simulink model "AIN_3x_3VT"  (R2018b)
settings: Solver=ode23t  StartTime=0.0  StopTime=0.5  RelTol=1e-3
undefined symbols (not defined in the file): DiscIntNeverNeededParam, fout
libraries: powerlib x26, powerlib_meascontrol x4
settings Model: Creator=K2  LastModifiedBy=VID Company

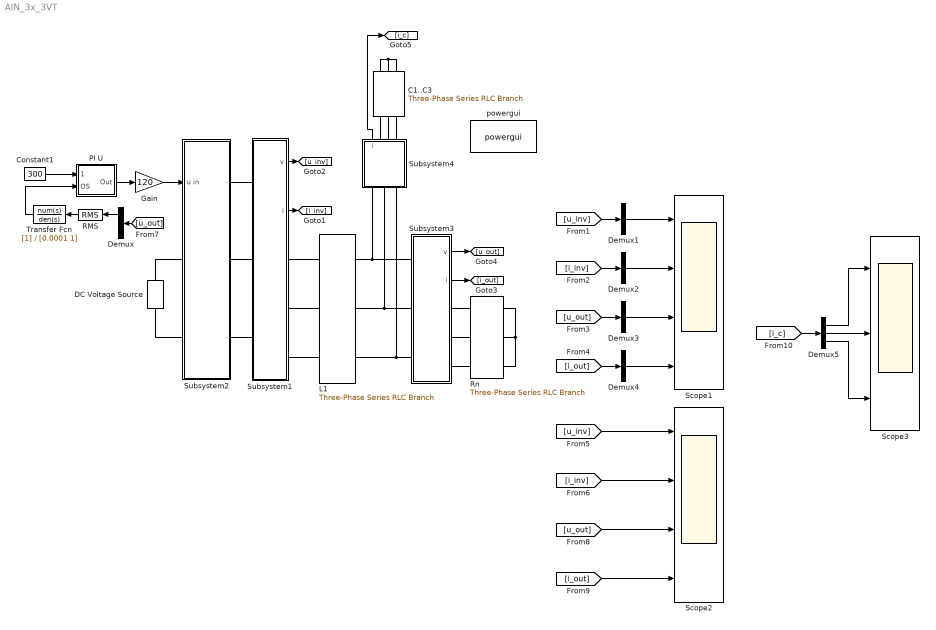
== system AIN_3x_3VT ==
  C1..C3 : powerlib/Elements/Three-Phase Series RLC Branch  LConnTagsString=A|B|C  RConnTagsString=A|B|C  BranchType=RC  Resistance=0.020  Inductance=1e-3  Capacitance=20e-6  Measurements=None
  Constant1 : Constant  Value=300  SampleTime=1e-6
  DC Voltage Source : powerlib/Electrical Sources/DC Voltage Source  Amplitude=550  Measurements=None
  Demux{,1..5} (6 alike) : Demux  Outputs=3
  Gain : Gain  Gain=120
  L1 : powerlib/Elements/Three-Phase Series RLC Branch  LConnTagsString=A|B|C  RConnTagsString=A|B|C  BranchType=RL  Resistance=0.2  Inductance=0.5e-3  Capacitance=1e-6  Measurements=None
  PI U : Subsystem
  RMS : powerlib_meascontrol/Measurements/RMS  TrueRMS=off  Freq=fout  RMSInit=0  Ts=0
  Rn : powerlib/Elements/Three-Phase Series RLC Branch  LConnTagsString=A|B|C  RConnTagsString=A|B|C  BranchType=RL  Resistance=10/sqrt(3)  Inductance=0.01e-3  Capacitance=1e-6  Measurements=None
  Scope1 : Scope  NumInputPorts=4
  Scope2 : Scope  NumInputPorts=4
  Scope3 : Scope  NumInputPorts=3
  Subsystem1 : Subsystem
  Subsystem2 : Subsystem
  Subsystem3 : Subsystem
  Subsystem4 : Subsystem
  Transfer Fcn : TransferFcn  Denominator=[0.0001 1]
  powergui : powerlib/powergui  Priority=1  SimulationMode=Discrete  SampleTime=1e-7  frequency=60  Iterations=50  frequencyindice=0  Pbase=100e6  ErrMax=1e-4  UnitsV=kV  UnitsW=MW  buscounter=0  FunctionMessages=off  echomessages=off  EnableUseOfTLC=off  CurrentSourceSwitches=off  DisableSnubberDevices=off  DisableRonSwitches=off  DisableVfSwitches=off  DisplayEquations=off  SolverType=Tustin/Backward Euler (TBE)  Interpol=off  ExternalGateDelay=off  methode=off  Ts=100  x0status=blocks  SPID=on  SwTol=0  HookPort=off  RestoreLinks=warning  ResistiveCurrentMeasurement=off  Frange=[0:2:500]  Ylog=off  Xlog=on  ShowGrid=off  save=off  variable=ZData  structure=logsout  ZoomFFT=on  StartTime=0.4  cycles=5  DisplayStyle=1  fundamental=50  FreqAxis=off  MaxFrequency=20000  frequencyindicesteady=1  RmsSteady=1  display=off
  wires:
  Constant1/1 -> PI U/1(Zad)
  RMS/1 -> Transfer Fcn/1
  Gain/1 -> Subsystem2/1(u in)
  PI U/1(Out) -> Gain/1
  Transfer Fcn/1 -> PI U/2(OS)
  Subsystem1/2(i) -> [i_inv]
  Subsystem1/1(v) -> [u_inv]
  Subsystem3/1(v) -> [u_out]
  Subsystem3/2(i) -> [i_out]
  [u_out] -> Demux/1
  Demux/1 -> RMS/1
  [u_inv] -> Demux1/1
  Demux1/2 -> Scope1/1
  [i_inv] -> Demux2/1
  Demux2/2 -> Scope1/2
  [u_out] -> Demux3/1
  Demux3/2 -> Scope1/3
  [i_out] -> Demux4/1
  Demux4/2 -> Scope1/4
  [u_inv] -> Scope2/1
  [i_inv] -> Scope2/2
  [i_out] -> Scope2/4
  [u_out] -> Scope2/3
  Subsystem4/1(i) -> [i_c]
  [i_c] -> Demux5/1
  Demux5/2 -> Scope3/2
  Demux5/1 -> Scope3/1
  Demux5/3 -> Scope3/3
  connections:
  Subsystem3/LConn1 -- Subsystem4/LConn1 -- L1/RConn1
  Subsystem3/LConn2 -- Subsystem4/LConn2 -- L1/RConn2
  Subsystem3/LConn3 -- Subsystem4/LConn3 -- L1/RConn3
  C1..C3/RConn1 -- C1..C3/RConn2 -- C1..C3/RConn3
  Rn/RConn1 -- Rn/RConn2 -- Rn/RConn3
  Subsystem2/RConn3 -- Subsystem1/LConn3
  Subsystem2/RConn1 -- Subsystem1/LConn1
  Subsystem2/RConn2 -- Subsystem1/LConn2
  Subsystem1/RConn1 -- L1/LConn1
  Subsystem1/RConn2 -- L1/LConn2
  Subsystem1/RConn3 -- L1/LConn3
  Subsystem3/RConn1 -- Rn/LConn1
  Subsystem3/RConn2 -- Rn/LConn2
  Subsystem3/RConn3 -- Rn/LConn3
  DC Voltage Source/RConn1 -- Subsystem2/LConn1
  DC Voltage Source/LConn1 -- Subsystem2/LConn2
  C1..C3/LConn1 -- Subsystem4/RConn1
  C1..C3/LConn2 -- Subsystem4/RConn2
  C1..C3/LConn3 -- Subsystem4/RConn3

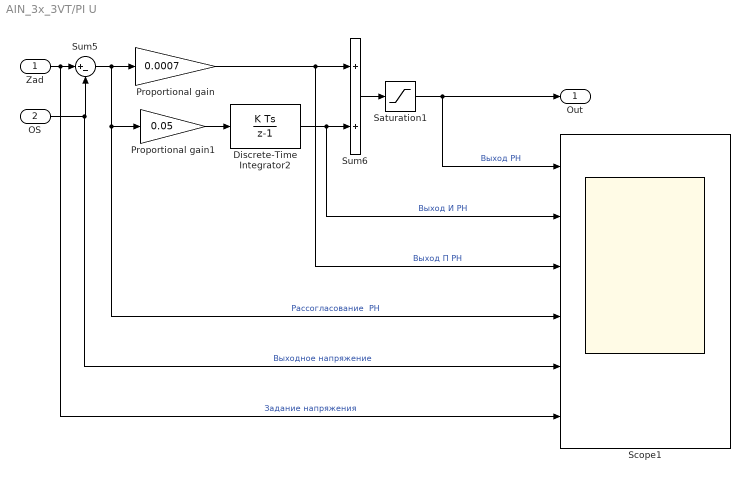
== system AIN_3x_3VT/PI U ==
  Zad : Inport
  OS : Inport  Port=2
  Discrete-Time Integrator2 : DiscreteIntegrator  SampleTime=-1  LimitOutput=on  UpperSaturationLimit=1  LowerSaturationLimit=0  ICPrevOutput=DiscIntNeverNeededParam  ICPrevScaledInput=DiscIntNeverNeededParam
  Proportional gain : Gain  Gain=0.0007  SaturateOnIntegerOverflow=on  OutDataTypeStr=Inherit: Same as input  ParamDataTypeStr=Inherit: Same as input
  Proportional gain1 : Gain  Gain=0.05  SaturateOnIntegerOverflow=on  OutDataTypeStr=Inherit: Same as input  ParamDataTypeStr=Inherit: Same as input
  Saturation1 : Saturate  UpperLimit=1  LowerLimit=0
  Scope1 : Scope  NumInputPorts=6
  Sum5 : Sum  Inputs=|+-  SaturateOnIntegerOverflow=on  InputSameDT=on  OutDataTypeStr=Inherit: Same as first input
  Sum6 : Sum  SaturateOnIntegerOverflow=on  InputSameDT=on  OutDataTypeStr=Inherit: Same as first input
  Out : Outport
  wires:
  Proportional gain/1 -> Scope1/3, Sum6/1  "Выход П РН"
  Discrete-Time Integrator2/1 -> Sum6/2, Scope1/2  "Выход И РН"
  OS/1 -> Scope1/5, Sum5/2  "Выходное напряжение"
  Zad/1 -> Scope1/6, Sum5/1  "Задание напряжения"
  Sum5/1 -> Proportional gain1/1, Scope1/4, Proportional gain/1  "Рассогласование  РН"
  Sum6/1 -> Saturation1/1
  Saturation1/1 -> Out/1, Scope1/1  "Выход РН"
  Proportional gain1/1 -> Discrete-Time Integrator2/1

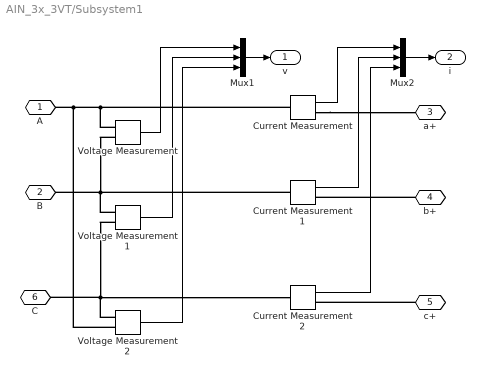
== system AIN_3x_3VT/Subsystem1 ==
  Current Measurement : powerlib/Measurements/Current Measurement  PhasorSimulation=off  OutputType=Complex  PSBequivalent=0
  Current Measurement1 : powerlib/Measurements/Current Measurement  PhasorSimulation=off  OutputType=Complex  PSBequivalent=0
  Current Measurement2 : powerlib/Measurements/Current Measurement  PhasorSimulation=off  OutputType=Complex  PSBequivalent=0
  Mux1 : Mux  Inputs=3
  Mux2 : Mux  Inputs=3
  Voltage Measurement : powerlib/Measurements/Voltage Measurement  PhasorSimulation=off  OutputType=Complex  PSBequivalent=0
  Voltage Measurement1 : powerlib/Measurements/Voltage Measurement  PhasorSimulation=off  OutputType=Complex  PSBequivalent=0
  Voltage Measurement2 : powerlib/Measurements/Voltage Measurement  PhasorSimulation=off  OutputType=Complex  PSBequivalent=0
  A : PMIOPort  Side=Left
  B : PMIOPort  Port=2  Side=Left
  a+ : PMIOPort  Port=3  Side=Right
  b+ : PMIOPort  Port=4  Side=Right
  c+ : PMIOPort  Port=5  Side=Right
  C : PMIOPort  Port=6  Side=Left
  v : Outport
  i : Outport  Port=2
  wires:
  Voltage Measurement1/1 -> Mux1/2
  Current Measurement2/1 -> Mux2/3
  Voltage Measurement2/1 -> Mux1/3
  Current Measurement/1 -> Mux2/1
  Voltage Measurement/1 -> Mux1/1
  Mux1/1 -> v/1
  Current Measurement1/1 -> Mux2/2
  Mux2/1 -> i/1
  connections:
  Current Measurement/RConn1 -- a+/RConn1
  Current Measurement/LConn1 -- Voltage Measurement/LConn1 -- Voltage Measurement2/LConn2 -- A/RConn1
  Voltage Measurement2/LConn1 -- C/RConn1 -- Voltage Measurement1/LConn2 -- Current Measurement2/LConn1
  c+/RConn1 -- Current Measurement2/RConn1
  Voltage Measurement/LConn2 -- B/RConn1 -- Current Measurement1/LConn1 -- Voltage Measurement1/LConn1
  b+/RConn1 -- Current Measurement1/RConn1

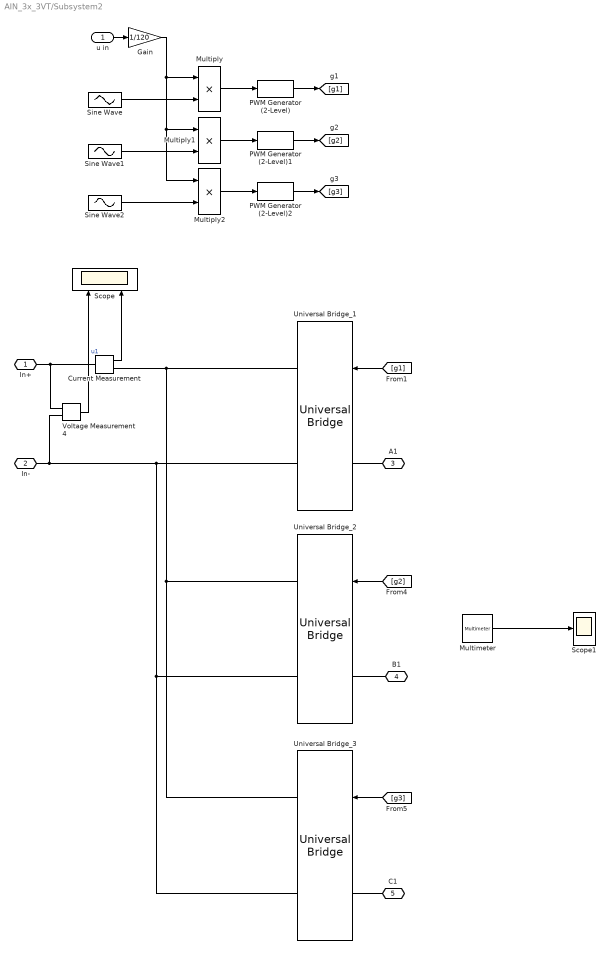
== system AIN_3x_3VT/Subsystem2 ==
  u in : Inport
  Current Measurement : powerlib/Measurements/Current Measurement  PhasorSimulation=off  OutputType=Complex  PSBequivalent=0
  Gain : Gain  Gain=1/120
  Multimeter : powerlib/Measurements/Multimeter  PhasorSimulation=off  OutputType=Complex  sel=[1 2]  L=2  Gain=[1 1]  yselected={'Isw1: Subsystem2/Universal Bridge_1','Isw2: Subsystem2/Universal Bridge_1'};  PSBOutputType=1  PSBequivalent=0  AxesSetting=[0,0.1,-100,100]  Display=0  SavedBlockNames=-11
  Multiply : Product
  Multiply1 : Product
  Multiply2 : Product
  PWM Generator (2-Level) : powerlib_meascontrol/Pulse & Signal Generators/PWM Generator (2-Level)  ModulatorType=Single-phase half-bridge (2 pulses)  ModulatorMode=Unsynchronized  Fc=fPWM  Pc=0  nF=27  MinMax="[ -1  1 ]"  SamplingTechnique=Symmetrical regular (single edge)  ModulatingSignals=off  m=0.8  Freq=60  Phase=0  Ts=0  ShowCarrierOutport=off
      settings: SourceProductName=Simscape Power Systems
  PWM Generator (2-Level)1 : powerlib_meascontrol/Pulse & Signal Generators/PWM Generator (2-Level)  ModulatorType=Single-phase half-bridge (2 pulses)  ModulatorMode=Unsynchronized  Fc=fPWM  Pc=0  nF=27  MinMax="[ -1  1 ]"  SamplingTechnique=Symmetrical regular (single edge)  ModulatingSignals=off  m=0.8  Freq=60  Phase=0  Ts=0  ShowCarrierOutport=off
      settings: SourceProductName=Simscape Power Systems
  PWM Generator (2-Level)2 : powerlib_meascontrol/Pulse & Signal Generators/PWM Generator (2-Level)  ModulatorType=Single-phase half-bridge (2 pulses)  ModulatorMode=Unsynchronized  Fc=fPWM  Pc=0  nF=27  MinMax="[ -1  1 ]"  SamplingTechnique=Symmetrical regular (single edge)  ModulatingSignals=off  m=0.8  Freq=60  Phase=0  Ts=0  ShowCarrierOutport=off
      settings: SourceProductName=Simscape Power Systems
  Scope : Scope  NumInputPorts=2
  Scope1 : Scope
  Sine Wave : Sin  Amplitude=0.99  Frequency=fout*2*pi  SampleTime=0
  Sine Wave1 : Sin  Amplitude=0.99  Frequency=fout*2*pi  Phase=2*pi*fout*(120/360)  SampleTime=0
  Sine Wave2 : Sin  Amplitude=0.99  Frequency=fout*2*pi  Phase=2*pi*fout*(240/360)  SampleTime=0
  Universal Bridge_1 : powerlib/Power Electronics/Universal Bridge  Arms=1  SnubberResistance=1e5  SnubberCapacitance=inf  Device=IGBT / Diodes  Ron=5e-3  Lon=0  ForwardVoltages="[  1.5  1  ]"  ForwardVoltage=0  GTOparameters=[ 10e-6 , 20e-6 ]  IGBTparameters=[ 1e-6 , 2e-6 ]  Measurements=Device currents  Measurements_2=None  converterType=Rectifier
  Universal Bridge_2 : powerlib/Power Electronics/Universal Bridge  Arms=1  SnubberResistance=1e5  SnubberCapacitance=inf  Device=IGBT / Diodes  Ron=5e-3  Lon=0  ForwardVoltages="[  1.5  1  ]"  ForwardVoltage=0  GTOparameters=[ 10e-6 , 20e-6 ]  IGBTparameters=[ 1e-6 , 2e-6 ]  Measurements=None  Measurements_2=None  converterType=Rectifier
  Universal Bridge_3 : powerlib/Power Electronics/Universal Bridge  Arms=1  SnubberResistance=1e5  SnubberCapacitance=inf  Device=IGBT / Diodes  Ron=5e-3  Lon=0  ForwardVoltages="[  1.5  1  ]"  ForwardVoltage=0  GTOparameters=[ 10e-6 , 20e-6 ]  IGBTparameters=[ 1e-6 , 2e-6 ]  Measurements=None  Measurements_2=None  converterType=Rectifier
  Voltage Measurement4 : powerlib/Measurements/Voltage Measurement  PhasorSimulation=off  OutputType=Complex  PSBequivalent=0
  In+ : PMIOPort  Side=Left
  In- : PMIOPort  Port=2  Side=Left
  A1 : PMIOPort  Port=3  Side=Right
  B1 : PMIOPort  Port=4  Side=Right
  C1 : PMIOPort  Port=5  Side=Right
  wires:
  PWM Generator (2-Level)/1 -> [g1]
  Gain/1 -> Multiply1/1, Multiply2/1, Multiply/1
  u in/1 -> Gain/1
  Multiply/1 -> PWM Generator (2-Level)/1
  Sine Wave/1 -> Multiply/2
  Current Measurement/1 -> Scope/2
  Voltage Measurement4/1 -> Scope/1  "u1"
  Multiply1/1 -> PWM Generator (2-Level)1/1
  Multiply2/1 -> PWM Generator (2-Level)2/1
  PWM Generator (2-Level)2/1 -> [g3]
  PWM Generator (2-Level)1/1 -> [g2]
  [g1] -> Universal Bridge_1/1
  [g2] -> Universal Bridge_2/1
  [g3] -> Universal Bridge_3/1
  Multimeter/1 -> Scope1/1
  Sine Wave1/1 -> Multiply1/2
  Sine Wave2/1 -> Multiply2/2
  connections:
  Current Measurement/LConn1 -- Voltage Measurement4/LConn1 -- In+/RConn1
  In-/RConn1 -- Voltage Measurement4/LConn2 -- Universal Bridge_3/RConn2 -- Universal Bridge_2/RConn2 -- Universal Bridge_1/RConn2
  Current Measurement/RConn1 -- Universal Bridge_2/RConn1 -- Universal Bridge_3/RConn1 -- Universal Bridge_1/RConn1
  A1/RConn1 -- Universal Bridge_1/LConn1
  B1/RConn1 -- Universal Bridge_2/LConn1
  C1/RConn1 -- Universal Bridge_3/LConn1

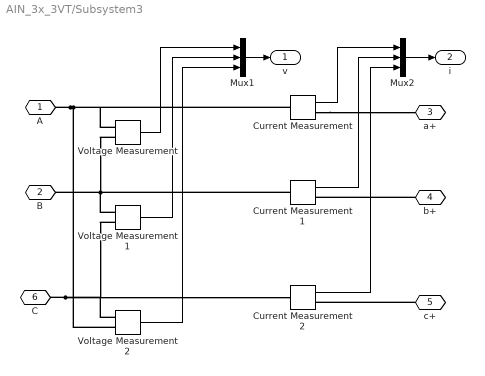
== system AIN_3x_3VT/Subsystem3 ==
  Current Measurement : powerlib/Measurements/Current Measurement  PhasorSimulation=off  OutputType=Complex  PSBequivalent=0
  Current Measurement1 : powerlib/Measurements/Current Measurement  PhasorSimulation=off  OutputType=Complex  PSBequivalent=0
  Current Measurement2 : powerlib/Measurements/Current Measurement  PhasorSimulation=off  OutputType=Complex  PSBequivalent=0
  Mux1 : Mux  Inputs=3
  Mux2 : Mux  Inputs=3
  Voltage Measurement : powerlib/Measurements/Voltage Measurement  PhasorSimulation=off  OutputType=Complex  PSBequivalent=0
  Voltage Measurement1 : powerlib/Measurements/Voltage Measurement  PhasorSimulation=off  OutputType=Complex  PSBequivalent=0
  Voltage Measurement2 : powerlib/Measurements/Voltage Measurement  PhasorSimulation=off  OutputType=Complex  PSBequivalent=0
  A : PMIOPort  Side=Left
  B : PMIOPort  Port=2  Side=Left
  a+ : PMIOPort  Port=3  Side=Right
  b+ : PMIOPort  Port=4  Side=Right
  c+ : PMIOPort  Port=5  Side=Right
  C : PMIOPort  Port=6  Side=Left
  v : Outport
  i : Outport  Port=2
  wires:
  Voltage Measurement1/1 -> Mux1/2
  Current Measurement2/1 -> Mux2/3
  Voltage Measurement2/1 -> Mux1/3
  Current Measurement/1 -> Mux2/1
  Voltage Measurement/1 -> Mux1/1
  Mux1/1 -> v/1
  Current Measurement1/1 -> Mux2/2
  Mux2/1 -> i/1
  connections:
  Current Measurement/RConn1 -- a+/RConn1
  A/RConn1 -- Current Measurement/LConn1 -- Voltage Measurement/LConn1 -- Voltage Measurement2/LConn2
  C/RConn1 -- Voltage Measurement2/LConn1 -- Current Measurement2/LConn1 -- Voltage Measurement1/LConn2
  c+/RConn1 -- Current Measurement2/RConn1
  Voltage Measurement/LConn2 -- Current Measurement1/LConn1 -- Voltage Measurement1/LConn1 -- B/RConn1
  b+/RConn1 -- Current Measurement1/RConn1

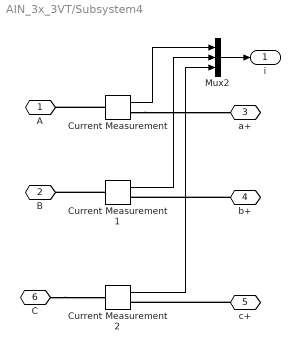
== system AIN_3x_3VT/Subsystem4 ==
  Current Measurement : powerlib/Measurements/Current Measurement  PhasorSimulation=off  OutputType=Complex  PSBequivalent=0
  Current Measurement1 : powerlib/Measurements/Current Measurement  PhasorSimulation=off  OutputType=Complex  PSBequivalent=0
  Current Measurement2 : powerlib/Measurements/Current Measurement  PhasorSimulation=off  OutputType=Complex  PSBequivalent=0
  Mux2 : Mux  Inputs=3
  A : PMIOPort  Side=Left
  B : PMIOPort  Port=2  Side=Left
  a+ : PMIOPort  Port=3  Side=Right
  b+ : PMIOPort  Port=4  Side=Right
  c+ : PMIOPort  Port=5  Side=Right
  C : PMIOPort  Port=6  Side=Left
  i : Outport
  wires:
  Current Measurement2/1 -> Mux2/3
  Current Measurement/1 -> Mux2/1
  Current Measurement1/1 -> Mux2/2
  Mux2/1 -> i/1
  connections:
  Current Measurement/RConn1 -- a+/RConn1
  Current Measurement/LConn1 -- A/RConn1
  C/RConn1 -- Current Measurement2/LConn1
  c+/RConn1 -- Current Measurement2/RConn1
  Current Measurement1/LConn1 -- B/RConn1
  b+/RConn1 -- Current Measurement1/RConn1
